simulink model "Quadcopter_Model"  (R2021a)
settings: Solver=VariableStepAuto  StartTime=0.0  StopTime=2  RelTol=1e-3
values from neighbouring files (symbols this model uses):
  h_des = 1    [quadcopter_data.m]
  K_z = 5    [quadcopter_data.m]
  quad_data = [      9.81,             0.063,            5.82857e-05,      7.16914e-05,      1.0e-04,          0.0624,           0.0107,           7.8264e-04,       1.15          ]    [quadcopter_data.m]
  y_init_conds = [      0,      0,      0,      0,      0,      0,      0,      0,      0   ]    [quadcopter_data.m]
settings Model: Creator=Utente  LastModifiedBy=Utente

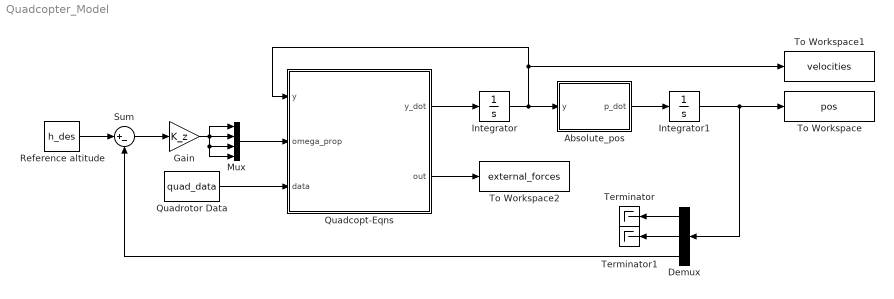
== system Quadcopter_Model ==
  Absolute_pos : MATLAB Function  TreatAsAtomicUnit=on
  Demux : Demux  Outputs=3
  Gain : Gain  Gain=K_z
  Integrator : Integrator  InitialCondition=y_init_conds
  Integrator1 : Integrator  InitialCondition=[0 0 0]
  Mux : Mux
  Quadcopt-Eqns : MATLAB Function  TreatAsAtomicUnit=on
  Quadrotor Data : Constant  Value=quad_data
  Reference altitude : Constant  Value=h_des
  Sum : Sum  Inputs=|+-
  Terminator : Terminator
  Terminator1 : Terminator
  To Workspace : ToWorkspace  VariableName=pos  SampleTime=-1
      settings: Save2DSignal=2-D array (concatenate along first dimension)
  To Workspace1 : ToWorkspace  VariableName=velocities  SampleTime=-1
      settings: Save2DSignal=2-D array (concatenate along first dimension)
  To Workspace2 : ToWorkspace  VariableName=external_forces  SampleTime=-1
      settings: Save2DSignal=2-D array (concatenate along first dimension)
  wires:
  Quadrotor Data/1 -> Quadcopt-Eqns/3(data)
  Quadcopt-Eqns/1(y_dot) -> Integrator/1
  Integrator/1 -> Absolute_pos/1(y), To Workspace1/1, Quadcopt-Eqns/1(y)
  Absolute_pos/1(p_dot) -> Integrator1/1
  Integrator1/1 -> Demux/1, To Workspace/1
  Quadcopt-Eqns/2(out) -> To Workspace2/1
  Mux/1 -> Quadcopt-Eqns/2(omega_prop)
  Sum/1 -> Gain/1
  Gain/1 -> Mux/4, Mux/3, Mux/1, Mux/2
  Reference altitude/1 -> Sum/1
  Demux/3 -> Sum/2
  Demux/1 -> Terminator/1
  Demux/2 -> Terminator1/1

== matlab function Quadcopter_Model/Absolute_pos ==
  data: y input; p_dot output
function p_dot = fcn(y)
    
    % Remapping================================
    u       = y(1);
    v       = y(2);
    w       = y(3);
    omega_x = y(4);
    omega_y = y(5);
    omega_z = y(6);
    phi     = y(7);
    theta   = y(8);
    psi     = y(9);
    
    %ode for absolute position (rhs)
    p_dot = [ ((sin(phi)*v + w*cos(phi))*sin(theta) + cos(theta)*u)*cos(psi) + sin(psi)*(sin(phi)*w - v*cos(phi)), ...
              ((sin(phi)*v + w*cos(phi))*sin(theta) + cos(theta)*u)*sin(psi) - cos(psi)*(sin(phi)*w - v*cos(phi)), ...
              w*cos(theta)*cos(phi) + v*cos(theta)*sin(phi) - u*sin(theta) ...
            ];

end

== matlab function Quadcopter_Model/Quadcopt-Eqns ==
  data: y input; omega_prop input; y_dot output; data input; out output
function [y_dot,out] = fcn(y,omega_prop,data)

    % y' = y_dot = rhs(y,u)
    % y = [u,v,w,omega_x,omega_y,omega_z,phi,theta,psi]
    % y(1) = u ....

    % Extract data from vector
    g   = data(1);
    m   = data(2);
    ixx = data(3);
    iyy = data(4);
    izz = data(5);
    L   = data(6);
    CT  = data(7);
    CQ  = data(8);
    rho = data(9);
        
    % Remapping================================
    u       = y(1);
    v       = y(2);
    w       = y(3);
    omega_x = y(4);
    omega_y = y(5);
    omega_z = y(6);
    phi     = y(7);
    theta   = y(8);
    psi     = y(9);

    % Extract angular velocities of propeller
    omega1 = omega_prop(1);
    omega2 = omega_prop(2);
    omega3 = omega_prop(3);
    omega4 = omega_prop(4);

    % External force model=====================
    %Thrust forces of propeller
    ft1 = rho*CT*omega1^2;
    ft2 = rho*CT*omega2^2;
    ft3 = rho*CT*omega3^2;
    ft4 = rho*CT*omega4^2;

    %Drag torques of propeller
    tauD1 = +rho*CQ*omega1^2;
    tauD2 = -rho*CQ*omega2^2;
    tauD3 = +rho*CQ*omega3^2;
    tauD4 = -rho*CQ*omega4^2;

    %Aerodynamic drag + wind
    %TO ADD LATER ON...

    % Equations angular velocities
    

    % Rhs equations of Newton-Euler============
    y_dot = [ ...
             sin(theta)*g + v*omega_z - w*omega_y,...
             -sin(phi)*cos(theta)*g - u*omega_z + w*omega_x ,...
             -0.1e1/m*(cos(phi)*cos(theta)*g*m + v*omega_x*m - u*omega_y*m - ft1 - ft3 - ft4 - ft2),...
             (iyy - izz)*omega_z/ixx*omega_y - L*(ft2 - ft4)/ixx ,...
             (izz - ixx)*omega_z/iyy*omega_x - L*(ft1 - ft3)/iyy,...
             (omega_y*(ixx - iyy)*omega_x + tauD1 + tauD2 + tauD3 + tauD4)/izz,...
             (sin(theta)*omega_z*cos(phi) + sin(theta)*omega_y*sin(phi) + omega_x*cos(theta))/cos(theta),...
             -omega_z*sin(phi) + omega_y*cos(phi),...
             (omega_z*cos(phi) + omega_y*sin(phi))/cos(theta) ...
            ];

    % Export values of external forces
    out = [ft1,ft2,ft3,ft4,tauD1,tauD2,tauD3,tauD4];

end
